simulink model "blocks-simulink"  (R2024a)
settings: Solver=VariableStepAuto  StartTime=0.0  StopTime=10.0  RelTol=1e-3
settings Model: Creator=AULAS FCMN  LastModifiedBy=oel

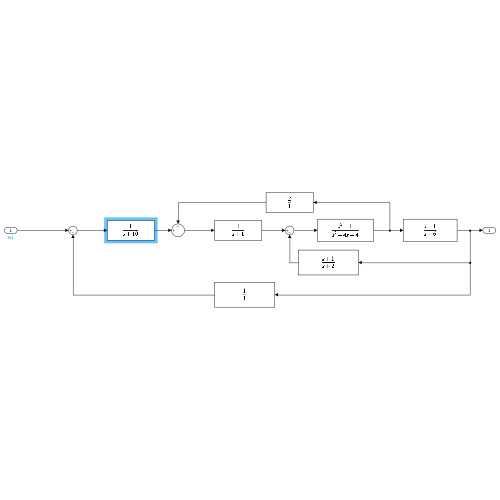
[thumbnail: Simulink's stored preview of the top-level diagram]
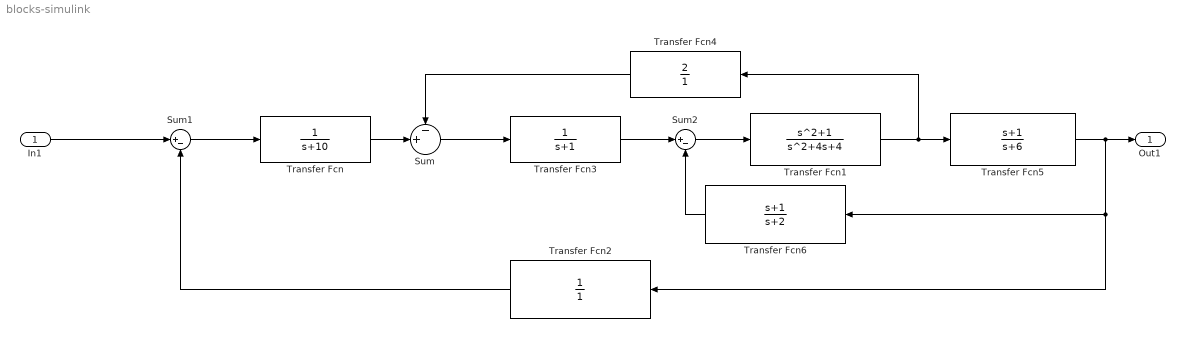
== system blocks-simulink ==
  In1 : Inport
  Sum : Sum  Inputs=-+|  CollapseMode=Specified dimension  RndMeth=Round
  Sum1 : Sum  Inputs=|+-
  Sum2 : Sum  Inputs=|+-
  Transfer Fcn : TransferFcn  Denominator=[1 10]
  Transfer Fcn1 : TransferFcn  Numerator=[1 0 1]  Denominator=[1 4 4 ]
  Transfer Fcn2 : TransferFcn  Denominator=[1]
  Transfer Fcn3 : TransferFcn  Denominator=[1 1]
  Transfer Fcn4 : TransferFcn  Numerator=[2]  Denominator=[1]
  Transfer Fcn5 : TransferFcn  Numerator=[1 1]  Denominator=[1 6]
  Transfer Fcn6 : TransferFcn  Numerator=[1 1]  Denominator=[1 2]
  Out1 : Outport
  wires:
  In1/1 -> Sum1/1
  Sum1/1 -> Transfer Fcn/1
  Transfer Fcn/1 -> Sum/2
  Sum/1 -> Transfer Fcn3/1
  Transfer Fcn4/1 -> Sum/1
  Transfer Fcn3/1 -> Sum2/1
  Sum2/1 -> Transfer Fcn1/1
  Transfer Fcn5/1 -> Transfer Fcn2/1, Transfer Fcn6/1, Out1/1
  Transfer Fcn2/1 -> Sum1/2
  Transfer Fcn6/1 -> Sum2/2
  Transfer Fcn1/1 -> Transfer Fcn5/1, Transfer Fcn4/1
